simulink model "TIntkVUs_DD"  (R2016b)
settings: configuration reference "CodeGenConfigSet" (kept outside this file)
values from neighbouring files (symbols this model uses):
  Air_tiSRCMaxTIntkVUsDefDeb_C = Calibration.Parameter    [init_TIntkVUs_DD.m]
  Air_tiSRCMaxTIntkVUsOKDeb_C = Calibration.Parameter    [init_TIntkVUs_DD.m]
  Air_tiSRCMinTIntkVUsDefDeb_C = Calibration.Parameter    [init_TIntkVUs_DD.m]
  Air_tiSRCMinTIntkVUsOKDeb_C = Calibration.Parameter    [init_TIntkVUs_DD.m]
  Air_tTransfTIntkVUs_CUR = Calibration.Parameter    [init_TIntkVUs_DD.m]
  Air_tTransfTIntkVUs_CURX = Calibration.Parameter    [init_TIntkVUs_DD.m]
  Air_uSRCTIntkVUsMax_C = Calibration.Parameter    [init_TIntkVUs_DD.m]
  Air_uSRCTIntkVUsMin_C = Calibration.Parameter    [init_TIntkVUs_DD.m]
undefined symbols (not defined in the file or in its folder): TIntkVUs_DD_DT
libraries: CXLib x6
settings Model: Creator=GaberXu  LastModifiedBy=wangrui
settings ConfigSetRef: SourceLocation=Base Workspace

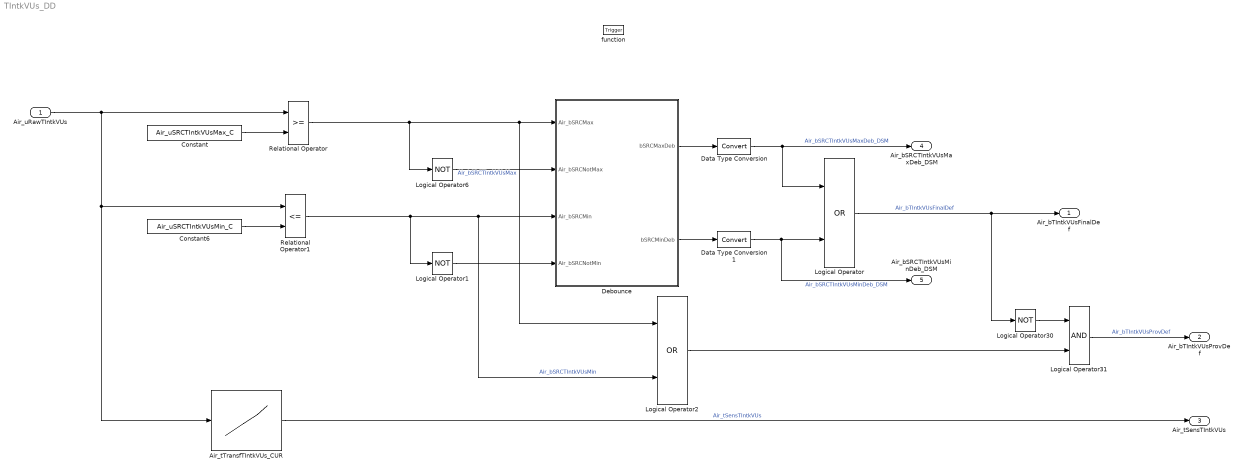
== system TIntkVUs_DD ==
  Air_uRawTIntkVUs : Inport  Tag=mv  Description=Raw ADC value of air temperature upstream of the intake valve  OutMin=0  OutMax=5000  OutDataTypeStr=Ad_mv
  function : TriggerPort  TriggerType=function-call  VariantControl=Variant
  Air_tTransfTIntkVUs_CUR : Lookup_n-D  NumberOfTableDimensions=1  BreakpointsForDimension1=Air_tTransfTIntkVUs_CURX  IndexSearchMethod=Linear search  BeginIndexSearchUsingPreviousIndexResult=on  UseOneInputPortForAllInputData=on  Table=Air_tTransfTIntkVUs_CUR  ExtrapMethod=Clip  UseLastTableValue=on  InternalRulePriority=Speed  OutDataTypeStr=Inherit: Inherit via back propagation  SaturateOnIntegerOverflow=on
  Constant : Constant  Value=Air_uSRCTIntkVUsMax_C
  Constant6 : Constant  Value=Air_uSRCTIntkVUsMin_C
  Data Type Conversion : DataTypeConversion
  Data Type Conversion1 : DataTypeConversion
  Debounce : Subsystem
  Logical Operator : Logic  Operator=OR  AllPortsSameDT=off  OutDataTypeStr=boolean
  Logical Operator1 : Logic  Operator=NOT  AllPortsSameDT=off  OutDataTypeStr=boolean
  Logical Operator2 : Logic  Operator=OR  AllPortsSameDT=off  OutDataTypeStr=boolean
  Logical Operator30 : Logic  Operator=NOT  AllPortsSameDT=off  OutDataTypeStr=boolean
  Logical Operator31 : Logic  AllPortsSameDT=off  OutDataTypeStr=boolean
  Logical Operator6 : Logic  Operator=NOT  AllPortsSameDT=off  OutDataTypeStr=boolean
  Relational Operator : RelationalOperator  OutDataTypeStr=boolean  RndMeth=Nearest  InputSameDT=on
  Relational Operator1 : RelationalOperator  Operator=<=  OutDataTypeStr=boolean  RndMeth=Nearest  InputSameDT=on
  Air_bTIntkVUsFinalDef : Outport  Description=Final defect of the raw air temperature upstream of the intake valve  OutMin=0  OutMax=1  OutDataTypeStr=boolean
  Air_bTIntkVUsProvDef : Outport  Description=Provisional defect of the raw air temperature upstream of the intake valve  Port=2  OutMin=0  OutMax=1  OutDataTypeStr=boolean
  Air_tSensTIntkVUs : Outport  Tag=deg  Description=Sensed value of air temperature upstream of the intake valve  Port=3  OutMin=-200  OutMax=200  OutDataTypeStr=Temp_deg
  Air_bSRCTIntkVUsMaxDeb_DSM : Outport  Description=DSM defect which the raw air temperature upstream of the intake valve is exceeding the maximum in SRC  Port=4  OutMin=0  OutMax=1  OutDataTypeStr=boolean
  Air_bSRCTIntkVUsMinDeb_DSM : Outport  Description=DSM defect which the raw air temperature upstream of the intake valve is exceeding the minimum in SRC  Port=5  OutMin=0  OutMax=1  OutDataTypeStr=boolean
  wires:
  Air_tTransfTIntkVUs_CUR/1 -> Air_tSensTIntkVUs/1  "Air_tSensTIntkVUs"
  Air_uRawTIntkVUs/1 -> Relational Operator/1, Air_tTransfTIntkVUs_CUR/1, Relational Operator1/1
  Constant/1 -> Relational Operator/2
  Relational Operator/1 -> Logical Operator6/1, Logical Operator2/1, Debounce/1(Air_bSRCMax)  "Air_bSRCTIntkVUsMax"
  Constant6/1 -> Relational Operator1/2
  Relational Operator1/1 -> Logical Operator1/1, Logical Operator2/2, Debounce/3(Air_bSRCMin)  "Air_bSRCTIntkVUsMin"
  Debounce/1(bSRCMaxDeb) -> Data Type Conversion/1
  Debounce/2(bSRCMinDeb) -> Data Type Conversion1/1
  Logical Operator/1 -> Logical Operator30/1, Air_bTIntkVUsFinalDef/1  "Air_bTIntkVUsFinalDef"
  Logical Operator6/1 -> Debounce/2(Air_bSRCNotMax)
  Logical Operator1/1 -> Debounce/4(Air_bSRCNotMin)
  Data Type Conversion/1 -> Air_bSRCTIntkVUsMaxDeb_DSM/1, Logical Operator/1  "Air_bSRCTIntkVUsMaxDeb_DSM"
  Data Type Conversion1/1 -> Air_bSRCTIntkVUsMinDeb_DSM/1, Logical Operator/2  "Air_bSRCTIntkVUsMinDeb_DSM"
  Logical Operator30/1 -> Logical Operator31/1
  Logical Operator2/1 -> Logical Operator31/2
  Logical Operator31/1 -> Air_bTIntkVUsProvDef/1  "Air_bTIntkVUsProvDef"

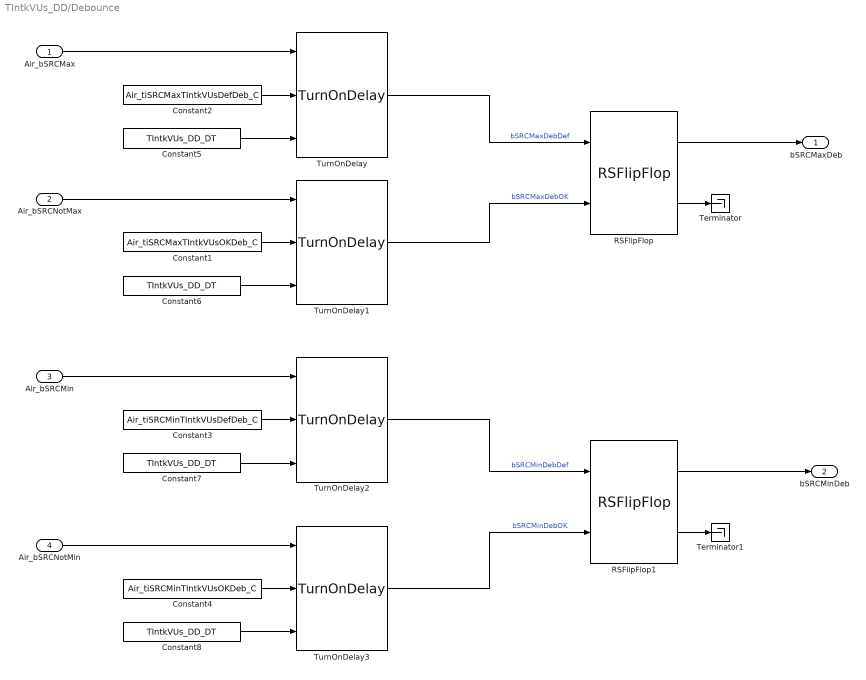
== system TIntkVUs_DD/Debounce ==
  Air_bSRCMax : Inport
  Air_bSRCNotMax : Inport  Port=2
  Air_bSRCMin : Inport  Port=3
  Air_bSRCNotMin : Inport  Port=4
  Constant1 : Constant  Value=Air_tiSRCMaxTIntkVUsOKDeb_C
  Constant2 : Constant  Value=Air_tiSRCMaxTIntkVUsDefDeb_C
  Constant3 : Constant  Value=Air_tiSRCMinTIntkVUsDefDeb_C
  Constant4 : Constant  Value=Air_tiSRCMinTIntkVUsOKDeb_C
  Constant{5..8} (4 alike) : Constant  Value=TIntkVUs_DD_DT
  RSFlipFlop : CXLib/RSFlipFlop
  RSFlipFlop1 : CXLib/RSFlipFlop
  Terminator : Terminator
  Terminator1 : Terminator
  TurnOnDelay{,1..3} (4 alike) : CXLib/TurnOnDelay
  bSRCMaxDeb : Outport
  bSRCMinDeb : Outport  Port=2
  wires:
  Constant8/1 -> TurnOnDelay3/3
  Constant7/1 -> TurnOnDelay2/3
  Constant6/1 -> TurnOnDelay1/3
  Constant5/1 -> TurnOnDelay/3
  Air_bSRCMax/1 -> TurnOnDelay/1
  RSFlipFlop1/2 -> Terminator1/1
  RSFlipFlop/2 -> Terminator/1
  Constant4/1 -> TurnOnDelay3/2
  TurnOnDelay3/1 -> RSFlipFlop1/2  "bSRCMinDebOK"
  Air_bSRCNotMin/1 -> TurnOnDelay3/1
  TurnOnDelay2/1 -> RSFlipFlop1/1  "bSRCMinDebDef"
  Air_bSRCMin/1 -> TurnOnDelay2/1
  Air_bSRCNotMax/1 -> TurnOnDelay1/1
  TurnOnDelay/1 -> RSFlipFlop/1  "bSRCMaxDebDef"
  Constant2/1 -> TurnOnDelay/2
  Constant1/1 -> TurnOnDelay1/2
  Constant3/1 -> TurnOnDelay2/2
  TurnOnDelay1/1 -> RSFlipFlop/2  "bSRCMaxDebOK"
  RSFlipFlop/1 -> bSRCMaxDeb/1
  RSFlipFlop1/1 -> bSRCMinDeb/1
